simulink model "remote"  (Simulink 7.6)
settings: Solver=ode5  StartTime=0.0  StopTime=10.0  FixedStep=Ts  RelTol=1e-3
values from neighbouring files (symbols this model uses):
  g = 9.8065    [kostas_malakies.mat]    (also in kostas_malakies2.mat; load_PMModel.m = 9.81; main.m; main_last.m)
  mass = 0.66    [kostas_malakies.mat]    (also in kostas_malakies2.mat; load_PMModel.m = 0.687; main_last.m)
  N = 5    [matlab.mat]
  Ts = 0.02    [kostas_malakies.mat]    (also in kostas_malakies2.mat; main.m; main_last.m; matlab.mat = 0.08)
  Ts_slow = 0.02    [kostas_malakies.mat]    (also in kostas_malakies2.mat; main.m; main_last.m)
  yaw0 = 0    [kostas_malakies.mat]    (also in kostas_malakies2.mat; main.m; main_last.m; matlab.mat = -0.0873)
undefined symbols (not defined in the file or in its folder): AA_delay_x, AA_delay_y, AA_delay_yaw, AA_delay_z, BB_delay_x, BB_delay_y, BB_delay_yaw, BB_delay_z, betas_x, betas_y, betas_yaw, betas_z, delay_steps_x, delay_steps_y, delay_steps_yaw, delay_steps_z, i_min_cs_pre_rough_x, i_min_cs_pre_rough_y, i_min_cs_pre_rough_yaw, i_min_cs_pre_rough_z, kalmf_bias_x, kalmf_bias_y, kalmf_bias_z, L_x, L_y, L_yaw, L_z, LL_PP_x, LL_PP_y, LL_PP_yaw, LL_PP_z, LL_ref_PP_x, LL_ref_PP_y, LL_ref_PP_yaw, LL_ref_PP_z, MM_x, MM_y, MM_yaw, MM_z, PP_x, PP_y, PP_yaw, PP_z, TT_PP_x, TT_PP_y, TT_PP_yaw, TT_PP_z, V_max_x, V_max_y, V_max_yaw, V_max_z
libraries: simulink x18, Hqaud_model_LIB_SI x5, Hquad_control_LIB_SI x1
(part 2 of 2)

== matlab function pos controller1/yaw_correction/Embedded MATLAB Function ==
  data: roll input double; pitch input double; pitch_bias input double; roll_bias input double; roll_rot output double; yaw input double; pitch_rot output double; pitch_bias_rot output double; roll_bias_rot output double
function [roll_rot,pitch_rot,pitch_bias_rot,roll_bias_rot] = fcn(roll,pitch,pitch_bias,roll_bias,yaw)
%#eml


sin_yaw=sin(yaw);
cos_yaw=cos(yaw);

R=[cos_yaw, -sin_yaw; sin_yaw, cos_yaw]';

temp=R*[pitch;roll];
pitch_rot=temp(1);
roll_rot=temp(2);

temp=R*[pitch_bias;roll_bias];
pitch_bias_rot=temp(1);
roll_bias_rot=temp(2);

== matlab function pos controller1/decoupling and rotation/rotate_to_quat_frame/Embedded MATLAB Function ==
  data: yaw input double; pitch_rot output double; pitch_cmd input double; roll_cmd input double; pitch_bias input double; roll_bias input double; roll_rot output double; pitch_bias_rot output double; roll_bias_rot output double
function [pitch_rot,roll_rot, pitch_bias_rot,roll_bias_rot] = fcn(yaw, pitch_cmd, roll_cmd, pitch_bias, roll_bias)
% calculate the desired set angles, according to the derivation in chapter
% 5.1.3 ('Decoupled Position Control Approach')

sin_yaw=sin(yaw);
cos_yaw=cos(yaw);

R=[cos_yaw, -sin_yaw; sin_yaw, cos_yaw];

temp=R*[pitch_cmd;roll_cmd];
pitch_rot=temp(1);
roll_rot=temp(2);

temp=R*[pitch_bias;roll_bias];
pitch_bias_rot=temp(1);
roll_bias_rot=temp(2);
